simulink model "integration"  (R2018a)
settings: Solver=FixedStepAuto  StartTime=0.0  StopTime=10.0  FixedStep=0.01  RelTol=1e-6
settings Model: Creator=Wang Tianci  LastModifiedBy=Wang Tianci

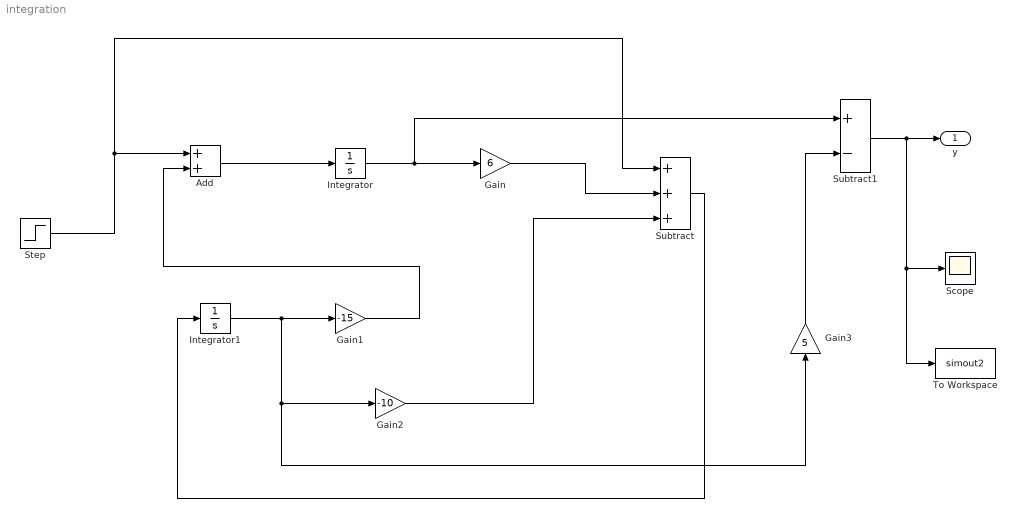
== system integration ==
  Add : Sum
  Gain : Gain  Gain=6
  Gain1 : Gain  Gain=-15
  Gain2 : Gain  Gain=-10
  Gain3 : Gain  Gain=5
  Integrator : Integrator  InitialCondition=1
  Integrator1 : Integrator
  Scope : Scope
  Step : Step  SampleTime=0
  Subtract : Sum  Inputs=+++
  Subtract1 : Sum  Inputs=+-
  To Workspace : ToWorkspace  VariableName=simout2  SampleTime=-1
  y : Outport
  wires:
  Gain2/1 -> Subtract/3
  Gain1/1 -> Add/2
  Add/1 -> Integrator/1
  Integrator1/1 -> Gain1/1, Gain2/1, Gain3/1
  Gain/1 -> Subtract/2
  Subtract/1 -> Integrator1/1
  Gain3/1 -> Subtract1/2
  Step/1 -> Add/1, Subtract/1
  Subtract1/1 -> y/1, Scope/1, To Workspace/1
  Integrator/1 -> Subtract1/1, Gain/1
